simulink model "simulation_of_spring_model"  (R2021a)
settings: Solver=VariableStepAuto  StartTime=0.0  StopTime=20  RelTol=1e-3
InitFcn:
  | m=1
  | k=10
  | b=0.4
libraries: simulink x1
settings Model: Creator=DELL  LastModifiedBy=DELL

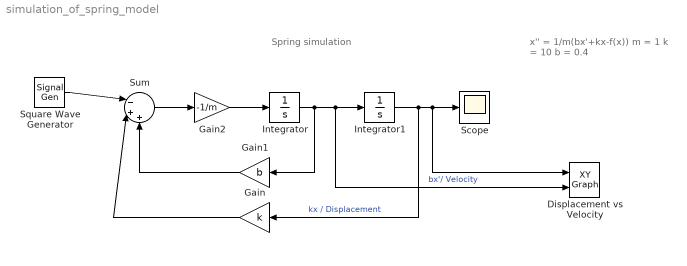
== system simulation_of_spring_model ==
  note: Spring simulation
  note: x'' = 1/m(bx'+kx-f(x))
      | m = 1
      | k = 10
      | b = 0.4
  Displacement vs Velocity : simulink/Sinks/XY Graph  xmin=-400  xmax=400  ymin=-600  ymax=600  st=-1
  Gain : Gain  Gain=k
  Gain1 : Gain  Gain=b
  Gain2 : Gain  Gain=-1/m
  Integrator : Integrator
  Integrator1 : Integrator
  Scope : Scope
  Square Wave Generator : SignalGenerator  WaveForm=square  Amplitude=200  Frequency=0.5
  Sum : Sum  Inputs=|-++
  wires:
  Integrator1/1 -> Displacement vs Velocity/1, Scope/1, Gain/1  "kx / Displacement"
  Integrator/1 -> Gain1/1, Displacement vs Velocity/2, Integrator1/1  "bx'/ Velocity"
  Sum/1 -> Gain2/1
  Square Wave Generator/1 -> Sum/1
  Gain1/1 -> Sum/3
  Gain/1 -> Sum/2
  Gain2/1 -> Integrator/1
